simulink library "FirDown"  (R2022b)
settings: Solver=VariableStepAuto  StartTime=0.0  StopTime=10.0  RelTol=1e-3
undefined symbols (not defined in the file or in its folder): Breed, designMultirateFIR
libraries: HandyTextFile x6, RTC x2, FeaturePath x1, dspmlti4 x1, FirGeneric x1, $bdroot x1
settings Model: Creator=jb10849  LastModifiedBy=fz1054048
settings SolverCC: AlgebraicLoopSolver=TrustRegion
settings DebuggingCC: UnconnectedInputMsg=warning  UnconnectedOutputMsg=warning  UnconnectedLineMsg=warning  SFMachineParentedDataDiag=warning  ArithmeticOperatorsInVariantConditions=warning
settings ModelReferenceCC: EnableRefExpFcnMdlSchedulingChecks=on
settings SFSimCC: SimUseLocalCustomCode=off  CustomCodeUndefinedFunction=UseInterfaceOnly
settings RTWCC: RTWUseLocalCustomCode=off  DLArmComputeVersion=19.05
settings CodeAppCC: StateflowObjectComments=on

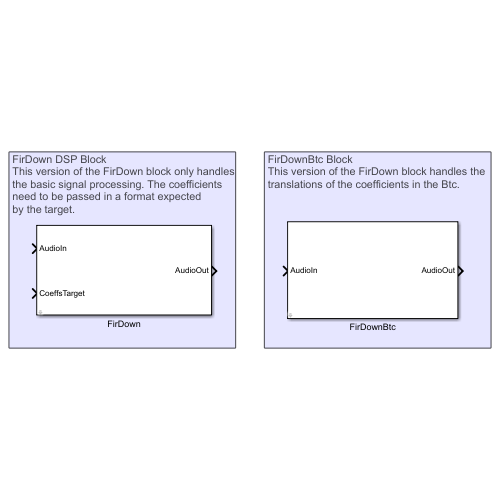
[thumbnail: Simulink's stored preview of the top-level diagram]
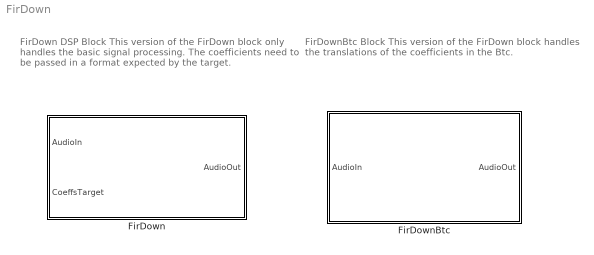
== system FirDown ==
  note: FirDown DSP Block
      | This version of the FirDown block only handles
      | the basic signal processing. The coefficients
      | need to be passed in a format expected
      | by the target.
  note: FirDownBtc Block
      | This version of the FirDown block handles the
      | translations of the coefficients in the Btc.
  FirDown : Subsystem  mask(Blocklib FirDown){Config=[], FeatureName=FirDown}
      mask prompts: Config "FirDownConfig"; FeatureName "Feature path name:"
      mask help:
      | See "help" or
      | run command
      | >> help FirDownConfig
      mask init:
      | blkh=gcbh;
      | Config=BTConfig.Assert(blkh,Config);
      | 
      | Config.Validate();
      | Config.DoMaskInit(blkh);
      mask Help: eval('help FirDownConfig')
      mask TypeOptions FeatureName: FeaturePath/FeatureName
      mask DialogControl ParamterGroupVar Prompt: Parameters
  FirDownBtc : Subsystem  mask(Blocklib FirDownBtc){Config=[], FeatureName=FirDownBtc}
      mask prompts: Config "FirDownBtcConfig"; FeatureName "Feature path name:"
      mask init:
      | blkh=gcbh;
      | Config=BTConfig.Assert(blkh,Config);
      | 
      | Config.Validate();
      | Config.DoMaskInit(blkh);
      mask TypeOptions FeatureName: FirDown/FeatureName

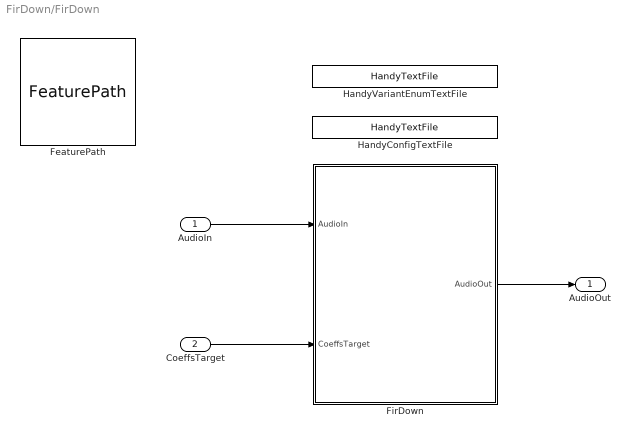
== system FirDown/FirDown ==
  AudioIn : Inport
  CoeffsTarget : Inport  Port=2
  FeaturePath : FeaturePath/FeaturePath  FeatureName=FirDown  IsGroup=off  GroupNumber=-1  IsModule=off  TriggerInit=[125 24 240 131]
      settings: SourceProductName=Bose Talaria
  FirDown : Subsystem  Variant=on
  HandyConfigTextFile : HandyTextFile/HandyTextFile  TemplateSource=Config  FileSuffix=File  OpenDialogOnLoad=off  UseThisBlockName=off  AddGrandParentNamePrefix=off  TheDefaultText=% $(FILENAME) $(PREFIX) $(SUFFIX)  ShowInLibBrowser=on
      settings: SourceProductName=Bose Talaria
  HandyVariantEnumTextFile : HandyTextFile/HandyTextFile  TemplateSource=<dialog fields>  FileSuffix=BreedEnum  OpenDialogOnLoad=off  UseThisBlockName=off  AddGrandParentNamePrefix=off  TheDefaultText=% $(FILENAME) $(PREFIX) $(SUFFIX)  ShowInLibBrowser=on
      settings: SourceProductName=Bose Talaria
  AudioOut : Outport
  wires:
  FirDown/1(AudioOut) -> AudioOut/1
  CoeffsTarget/1 -> FirDown/2(CoeffsTarget)
  AudioIn/1 -> FirDown/1(AudioIn)

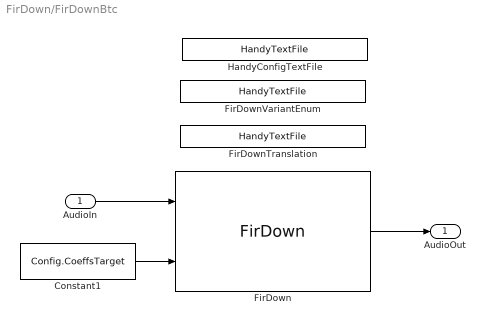
== system FirDown/FirDownBtc ==
  AudioIn : Inport
  Constant1 : Constant  Value=Config.CoeffsTarget  VectorParams1D=off  OutDataTypeStr=single
  FirDown : $bdroot/FirDown  Config=Config  FeatureName=FirDownBtc
  FirDownTranslation : HandyTextFile/HandyTextFile  TemplateSource=<dialog fields>  FileSuffix=File  OpenDialogOnLoad=off  UseThisBlockName=on  AddGrandParentNamePrefix=off  TheDefaultText=% $(FILENAME) $(PREFIX) $(SUFFIX)  ShowInLibBrowser=on
      settings: SourceProductName=Bose Talaria
  FirDownVariantEnum : HandyTextFile/HandyTextFile  TemplateSource=<dialog fields>  FileSuffix=VariantEnum  OpenDialogOnLoad=off  UseThisBlockName=on  AddGrandParentNamePrefix=off  TheDefaultText=% $(FILENAME) $(PREFIX) $(SUFFIX)  ShowInLibBrowser=on
      settings: SourceProductName=Bose Talaria
  HandyConfigTextFile : HandyTextFile/HandyTextFile  TemplateSource=Config  FileSuffix=File  OpenDialogOnLoad=off  UseThisBlockName=off  AddGrandParentNamePrefix=off  TheDefaultText=% $(FILENAME) $(PREFIX) $(SUFFIX)  ShowInLibBrowser=on
      settings: SourceProductName=Bose Talaria
  AudioOut : Outport
  wires:
  AudioIn/1 -> FirDown/1
  FirDown/1 -> AudioOut/1
  Constant1/1 -> FirDown/2

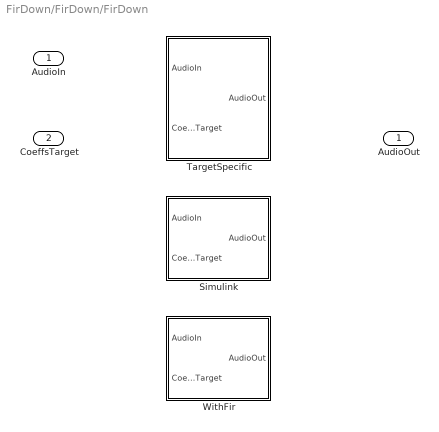
== system FirDown/FirDown/FirDown ==
  AudioIn : Inport
  CoeffsTarget : Inport  Port=2
  Simulink : Subsystem  VariantControl=Config.Breed == AsdHwEnum.Simulink
  TargetSpecific : Subsystem  VariantControl=(false)
  WithFir : Subsystem  VariantControl=(default)
      settings: LibrarySourceBlock=FirDown/FirDown/FirDown/Simulink
  AudioOut : Outport

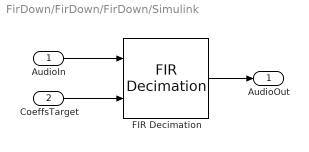
== system FirDown/FirDown/FirDown/Simulink ==
  AudioIn : Inport
  CoeffsTarget : Inport  Port=2
  FIR Decimation : dspmlti4/FIR Decimation  FilterSource=Input port  h=designMultirateFIR(1,2)  D=Config.DownFactor  filtStruct=Direct form  FilterObject=FDECIM  InputProcessing=Columns as channels (frame based)  framing=Enforce single-rate processing  AllowArbitraryInputLength=off  inputOffset=0  outputBufInitCond=0  roundingMode=Floor  overflowMode=off  firstCoeffDataTypeStr=Inherit: Same word length as input  firstCoeffMin=[]  firstCoeffMax=[]  firstCoeffLastDataTypeStr=Inherit: Same word length as input  outputDataTypeStr=Inherit: Same as accumulator  outputMin=[]  outputMax=[]  outputLastDataTypeStr=Inherit: Same as accumulator
      settings: LibrarySourceBlock=|
      | dsphdlsupportfiltering/FIR
      | Decimation
  AudioOut : Outport
  wires:
  AudioIn/1 -> FIR Decimation/1
  FIR Decimation/1 -> AudioOut/1
  CoeffsTarget/1 -> FIR Decimation/2

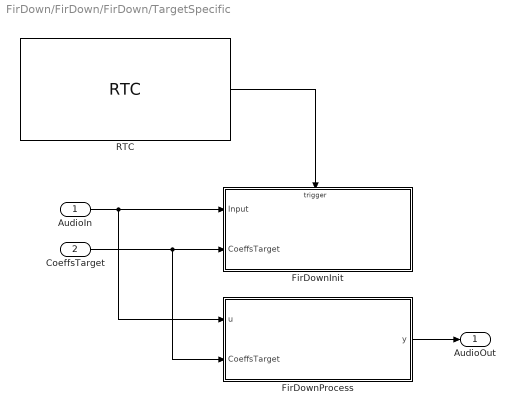
== system FirDown/FirDown/FirDown/TargetSpecific ==
  AudioIn : Inport
  CoeffsTarget : Inport  Port=2
  FirDownInit : MATLAB Function  TreatAsAtomicUnit=on  mask{DownFactor=Config.DownFactor, Breed=Config.Breed}
  FirDownProcess : MATLAB Function  TreatAsAtomicUnit=on  mask{UpFactor=Config.DownFactor, VariantUint8=Config.Breed}
  RTC : RTC/RTC  REQ_Priority=RTC_Mask.NormalPriority  RequestAtInit=on  EnableRequest=on  REQElemType1=uint32  REQElemWidth1=1  REQElemInitial1=[]  REQElemType2=uint32  REQElemWidth2=1  REQElemInitial2=[]  REQElemType3=uint32  REQElemWidth3=1  REQElemInitial3=[]  REQElemType4=uint32  REQElemWidth4=1  REQElemInitial4=[]  REQElemType5=uint32  REQElemWidth5=1  REQElemInitial5=[]  REQElemType6=uint32  REQElemWidth6=1  REQElemInitial6=[]  REQElemType7=uint32  REQElemWidth7=1  REQElemInitial7=[]  REQElemType8=uint32  REQElemWidth8=1  REQElemInitial8=[]  REQElemType9=uint32  REQElemWidth9=1  REQElemInitial9=[]  REQElemType10=uint32  REQElemWidth10=1  REQElemInitial10=[]  EnableResponse=off  EnableRSP_StatusIn=off  RSPElemType1=uint32  RSPElemWidth1=1  RSPElemType2=uint32  RSPElemWidth2=1  RSPElemType3=uint32  RSPElemWidth3=1  RSPElemType4=uint32  RSPElemWidth4=1  RSPElemType5=uint32  RSPElemWidth5=1  RSPElemType6=uint32  RSPElemWidth6=1  RSPElemType7=uint32  RSPElemWidth7=1  RSPElemType8=uint32  RSPElemWidth8=1  RSPElemType9=uint32  RSPElemWidth9=1  RSPElemType10=uint32  RSPElemWidth10=1  EnableNotification=off  EnableNTF_PrepTrig=off  NTFElemType1=uint32  NTFElemWidth1=1  NTFElemType2=uint32  NTFElemWidth2=1  NTFElemType3=uint32  NTFElemWidth3=1  NTFElemType4=uint32  NTFElemWidth4=1  NTFElemType5=uint32  NTFElemWidth5=1  NTFElemType6=uint32  NTFElemWidth6=1  NTFElemType7=uint32  NTFElemWidth7=1  NTFElemType8=uint32  NTFElemWidth8=1  NTFElemType9=uint32  NTFElemWidth9=1  NTFElemType10=uint32  NTFElemWidth10=1  MaskMessageName=InitReset
      settings: SourceProductName=Bose Talaria
  AudioOut : Outport
  wires:
  FirDownProcess/1(y) -> AudioOut/1
  RTC/1 -> FirDownInit/Trigger
  AudioIn/1 -> FirDownProcess/1(u), FirDownInit/1(Input)
  CoeffsTarget/1 -> FirDownProcess/2(CoeffsTarget), FirDownInit/2(CoeffsTarget)

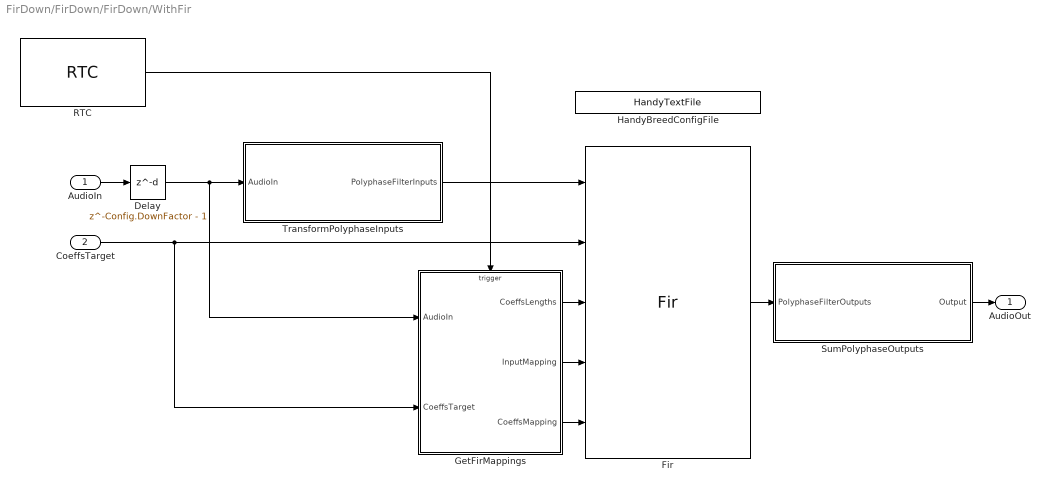
== system FirDown/FirDown/FirDown/WithFir ==
  AudioIn : Inport
  CoeffsTarget : Inport  Port=2
  Delay : Delay  DelayLength=Config.DownFactor - 1  InputProcessing=Columns as channels (frame based)
  Fir : FirGeneric/Fir  Config=Config.Fir  FeatureName=Fir
      settings: SourceProductName=Bose Blocklib
  GetFirMappings : MATLAB Function  TreatAsAtomicUnit=on  mask{DownFactor=Config.DownFactor}
  HandyBreedConfigFile : HandyTextFile/HandyTextFile  TemplateSource=<dialog fields>  FileSuffix=BreedConfig  OpenDialogOnLoad=off  UseThisBlockName=off  AddGrandParentNamePrefix=on  TheDefaultText=|  ShowInLibBrowser=on
      | % $(FILENAME) Setup model parameters for each "Init" callback (e.g. update diagram)
      | sample_rate_in_hertz = 44100;
      | frame_size = 32;
      | sysin_channel_count = 2;
      settings: SourceProductName=Bose Talaria
  RTC : RTC/RTC  REQ_Priority=RTC_Mask.NormalPriority  RequestAtInit=on  EnableRequest=on  REQElemType1=uint32  REQElemWidth1=1  REQElemInitial1=[]  REQElemType2=uint32  REQElemWidth2=1  REQElemInitial2=[]  REQElemType3=uint32  REQElemWidth3=1  REQElemInitial3=[]  REQElemType4=uint32  REQElemWidth4=1  REQElemInitial4=[]  REQElemType5=uint32  REQElemWidth5=1  REQElemInitial5=[]  REQElemType6=uint32  REQElemWidth6=1  REQElemInitial6=[]  REQElemType7=uint32  REQElemWidth7=1  REQElemInitial7=[]  REQElemType8=uint32  REQElemWidth8=1  REQElemInitial8=[]  REQElemType9=uint32  REQElemWidth9=1  REQElemInitial9=[]  REQElemType10=uint32  REQElemWidth10=1  REQElemInitial10=[]  EnableResponse=off  EnableRSP_StatusIn=off  RSPElemType1=uint32  RSPElemWidth1=1  RSPElemType2=uint32  RSPElemWidth2=1  RSPElemType3=uint32  RSPElemWidth3=1  RSPElemType4=uint32  RSPElemWidth4=1  RSPElemType5=uint32  RSPElemWidth5=1  RSPElemType6=uint32  RSPElemWidth6=1  RSPElemType7=uint32  RSPElemWidth7=1  RSPElemType8=uint32  RSPElemWidth8=1  RSPElemType9=uint32  RSPElemWidth9=1  RSPElemType10=uint32  RSPElemWidth10=1  EnableNotification=off  EnableNTF_PrepTrig=off  NTFElemType1=uint32  NTFElemWidth1=1  NTFElemType2=uint32  NTFElemWidth2=1  NTFElemType3=uint32  NTFElemWidth3=1  NTFElemType4=uint32  NTFElemWidth4=1  NTFElemType5=uint32  NTFElemWidth5=1  NTFElemType6=uint32  NTFElemWidth6=1  NTFElemType7=uint32  NTFElemWidth7=1  NTFElemType8=uint32  NTFElemWidth8=1  NTFElemType9=uint32  NTFElemWidth9=1  NTFElemType10=uint32  NTFElemWidth10=1  MaskMessageName=WithFirInitReset
      settings: SourceProductName=Bose Talaria
  SumPolyphaseOutputs : MATLAB Function  TreatAsAtomicUnit=on  mask{DownFactor=Config.DownFactor, FrameSizeIn=Config.FrameSizeIn, NumChannels=Config.NumChannels}
  TransformPolyphaseInputs : MATLAB Function  TreatAsAtomicUnit=on  mask{DownFactor=Config.DownFactor, FrameSizeIn=Config.FrameSizeIn, NumChannels=Config.NumChannels}
  AudioOut : Outport
  wires:
  AudioIn/1 -> Delay/1
  TransformPolyphaseInputs/1(PolyphaseFilterInputs) -> Fir/1
  CoeffsTarget/1 -> Fir/2, GetFirMappings/2(CoeffsTarget)
  RTC/1 -> GetFirMappings/Trigger
  GetFirMappings/1(CoeffsLengths) -> Fir/3
  GetFirMappings/2(InputMapping) -> Fir/4
  GetFirMappings/3(CoeffsMapping) -> Fir/5
  Fir/1 -> SumPolyphaseOutputs/1(PolyphaseFilterOutputs)
  SumPolyphaseOutputs/1(Output) -> AudioOut/1
  Delay/1 -> TransformPolyphaseInputs/1(AudioIn), GetFirMappings/1(AudioIn)

== matlab function FirDown/FirDown/TargetSpecific/FirDownProcess ==
  data: u input; y output; UpFactor parameter; Breed parameter; CoeffsTarget input
function y = FirDownProcess(u, UpFactor, Breed, CoeffsTarget)
% TO DO

y = u;
end

== matlab function FirDown/FirDown/WithFir/TransformPolyphaseInputs ==
  data: AudioIn input; PolyphaseFilterInputs output size=[FrameSizeIn/DownFactor NumChannels*DownFactor]; DownFactor parameter; FrameSizeIn parameter; NumChannels parameter
function PolyphaseFilterInputs = TransformPolyphaseInputs(AudioIn, DownFactor, FrameSizeIn, NumChannels)
% Converts standard filter inputs into polyphase filter inputs
%disp("Audio In ----------------------------------------------------")
%disp(AudioIn(:,1))
PolyphaseChannels = NumChannels*DownFactor;
PolyphaseFilterInputs = zeros(FrameSizeIn/DownFactor, PolyphaseChannels,'single');
for ch = 1:NumChannels
    for M = 1:DownFactor
        % Separation of single input into polyphase subfilter inputs 
        PolyphaseFilterInputs(:, (ch-1)*DownFactor+M) = AudioIn(M:DownFactor:FrameSizeIn, ch);
    end
end
%disp("Audio Out xxxxxxxxxxxxxxxxxxxxxxxxxxxxxxxxxxxxxxxxxxxxxxxxxxxx")
%disp(PolyphaseFilterInputs(:,1:4))
end

== matlab function FirDown/FirDown/TargetSpecific/FirDownInit ==
  data: Input input; DownFactor parameter; Breed parameter; CoeffsTarget input
  events: trigger input FUNCTION_CALL_EVENT
function FirDownInit(Input, DownFactor, Breed, CoeffsTarget)
% TODO
y = u;
end

== matlab function FirDown/FirDown/WithFir/SumPolyphaseOutputs ==
  data: PolyphaseFilterOutputs input; Output output size=[FrameSizeIn/DownFactor NumChannels]; DownFactor parameter; FrameSizeIn parameter; NumChannels parameter
function Output = SumPolyphaseOutputs(PolyphaseFilterOutputs, DownFactor, FrameSizeIn, NumChannels)
% Converts polyphase filter outputs into standard filter outputs

% Instantiate output array
Output = zeros(FrameSizeIn/DownFactor, NumChannels,'single');
for ch = 1: NumChannels
    % Summation of polyphase subfilter outputs into a single downsampled
    % output
    Output(:,ch) = sum(PolyphaseFilterOutputs(:,(ch-1)*DownFactor + (1:DownFactor)),2);
end
end

== matlab function FirDown/FirDown/WithFir/GetFirMappings ==
  data: AudioIn input; CoeffsTarget input; CoeffsLengths output; InputMapping output; CoeffsMapping output; DownFactor parameter
  events: trigger input FUNCTION_CALL_EVENT
function [CoeffsLengths, InputMapping, CoeffsMapping] = GetFirMappings(AudioIn, CoeffsTarget, DownFactor)

[~, NumChannels] = size(AudioIn);
NumOutputs = DownFactor*NumChannels;

% Coefficients are equally divided up into [DownFactor] number of coefficient
% sets. 
CoeffsLengths = uint32(ceil(ones(1,DownFactor).*(numel(CoeffsTarget)/DownFactor)));
% disp("CoeffsLengths -------------------------------------------------")
% disp(CoeffsLengths)


% Output is mapped as follows, where DownFactor = M and NumChannels = Nc
% ix = 0: Nc - 1
%   iy = 0: M - 1
% fcn(Input[ix], Filter[iy]) = Output[ix*M + iy]
%
% CoeffsMapping = [0, 1, 2 ... L-1, 0, 1, 2 ... L-1 ...]
CoeffsMapping = uint32(flip(mod(0:NumOutputs-1,DownFactor)));
% disp("CoeffsMappings -------------------------------------------------")
% disp(CoeffsMapping)
% InputMapping = [0, 1, 2, ... Nc-1]
InputMapping = uint32(0:NumOutputs-1);
% disp("InputMapping -------------------------------------------------")
% disp(InputMapping)

end
